simulink model "Modelo_Discreto_SS"  (R2019a)
settings: Solver=VariableStepAuto  StartTime=0.0  StopTime=500  RelTol=1e-3
model workspace (MAT data in the model file):
  P = [0.118997681558  0.340385726666  0.751267059306; 0.498364051982  0.58526775098  0.255095115459; 0.959743958516  0.223811939491  0.505957051665]
  xe = [0; 0; 0]
undefined symbols (not defined in the file or in its folder): sigbuilder_block
libraries: simulink x4
settings Model: OrderedModelArguments=off  Creator=Steven  LastModifiedBy=PC-88464
settings DataIOCC: ReturnWorkspaceOutputs=off
settings DebuggingCC: ArithmeticOperatorsInVariantConditions=warning
settings SFSimCC: SimUseLocalCustomCode=off
settings RTWCC: RTWUseLocalCustomCode=off
settings CodeAppCC: StateflowObjectComments=on

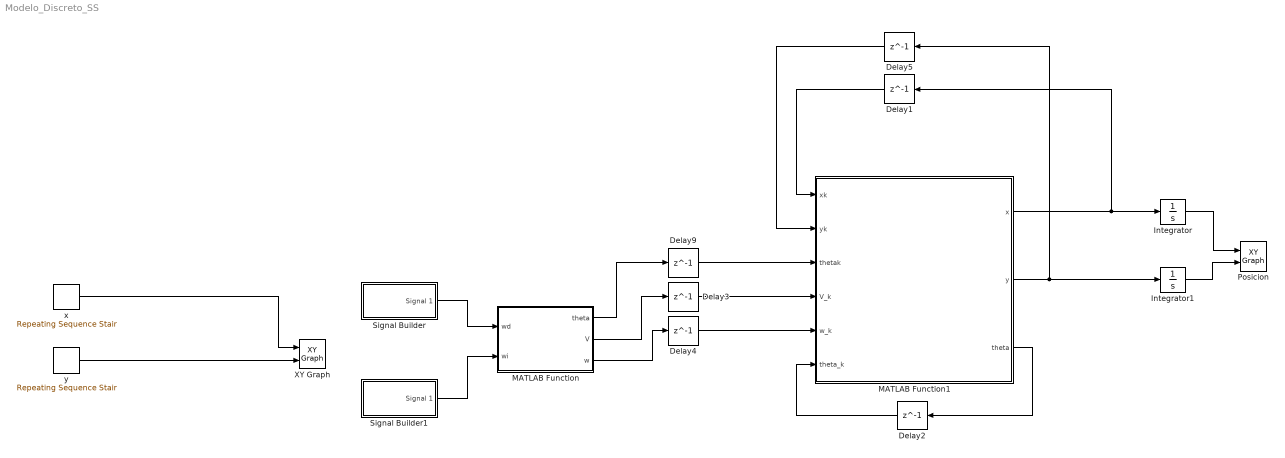
== system Modelo_Discreto_SS ==
  Delay{1..5,9} (6 alike) : Delay  DelayLength=1  InitialCondition=0  SampleTime=0.5
  Integrator : Integrator
  Integrator1 : Integrator
  MATLAB Function : MATLAB Function  TreatAsAtomicUnit=on
  MATLAB Function1 : MATLAB Function  TreatAsAtomicUnit=on  SystemSampleTime=0.5
  Posicion : simulink/Sinks/XY Graph  xmin=-2000  xmax=2000  ymin=-200  ymax=200  st=0.5
  Signal Builder : Subsystem  Tag=STV Subsys  LoadFcn=sigbuilder_block('load',[6 99 1012.5 413.25 ]);  StartFcn=sigbuilder_block('start');  StopFcn=sigbuilder_block('stop');  ClipboardFcn=sigbuilder_block('clipboard');  mask(Sigbuilder block){tuvar=[0:10]}
      mask help: Simulink:masks:SigbuilderBlock_MD
      mask init:
      | if ~strcmp(get_param(bdroot(gcbh),'SimulationStatus'),'stopped') tuvar = sigbuilder_block('maskInit'); end
      settings: CopyFcn=sigbuilder_block('copy');  DeleteFcn=sigbuilder_block('delete');  ModelCloseFcn=sigbuilder_block('modelClose');  PreSaveFcn=sigbuilder_block('preSave');  PauseFcn=sigbuilder_block('pause');  ContinueFcn=sigbuilder_block('continue');  NameChangeFcn=sigbuilder_block('namechange');  OpenFcn=sigbuilder_block('open',[51 123.75 1012.5 453.75 ]);  CloseFcn=sigbuilder_block('close');
      mask Display: plot(0, 0, 100, 100,[2, 2, 32, 32, 2], [68, 8, 8, 68, 68],[32, 2], [38, 38], [32, 19, 2],[53, 60, 44], [32, 17, 17, 2],[16, 16, 31, 31]);txt = getActiveGroup(gcbh);text(2, 100, txt,'verticalAlignment', 'top');
  Signal Builder1 : Subsystem  Tag=STV Subsys  LoadFcn=sigbuilder_block('load',[0.75 0.75 510.75 487.5 ]);  StartFcn=sigbuilder_block('start');  StopFcn=sigbuilder_block('stop');  ClipboardFcn=sigbuilder_block('clipboard');  mask(Sigbuilder block){tuvar=[0:10]}
      mask help: Simulink:masks:SigbuilderBlock_MD
      mask init:
      | if ~strcmp(get_param(bdroot(gcbh),'SimulationStatus'),'stopped') tuvar = sigbuilder_block('maskInit'); end
      settings: CopyFcn=sigbuilder_block('copy');  DeleteFcn=sigbuilder_block('delete');  ModelCloseFcn=sigbuilder_block('modelClose');  PreSaveFcn=sigbuilder_block('preSave');  PauseFcn=sigbuilder_block('pause');  ContinueFcn=sigbuilder_block('continue');  NameChangeFcn=sigbuilder_block('namechange');  OpenFcn=sigbuilder_block('open',[0.75 0.75 510.75 487.5 ]);  CloseFcn=sigbuilder_block('close');
      mask Display: plot(0, 0, 100, 100,[2, 2, 32, 32, 2], [68, 8, 8, 68, 68],[32, 2], [38, 38], [32, 19, 2],[53, 60, 44], [32, 17, 17, 2],[16, 16, 31, 31]);txt = getActiveGroup(gcbh);text(2, 100, txt,'verticalAlignment', 'top');
  XY Graph : simulink/Sinks/XY Graph  xmin=0  xmax=3000  ymin=0  ymax=200  st=-1
  x : simulink/Sources/Repeating Sequence Stair  OutValues="[0\t0\t0.122357536764706\t0.367004790785897\t0.733670540416495\t1.22188038737213\t1.83095716997706\t2.56002156384211\t3.40799286951678\t4.37358998651249\t5.45533257294931\t6.65154238993406\t7.96034482963452\t9.37967062587108\t10.9072577459058\t12.5074870935543\t14.1358531150623\t15.8024628907078\t17.5073781191743\t19.2506527356775\t21.0323328948846\t22.8524569547695\t24.6870589097060\t26.5315151793224\t28.3858216367550\t30.2499741436157\t32.1239685499954\t34.0078006944664\t35.9014664040855\t37.8049614943969\t39.7182817694354\t41.6414230217288\t43.5743810323012\t45.5171515706758\t47.4697303948779\t49.4321132514379\t51.4042958753942\t53.3862739902961\t55.3780433082071\t57.3795995297073\t59.3909383438971\t61.4055696132564\t63.4219031302490\t65.4399669647606\t67.4597607181438\t69.4812839897551\t71.5045363769553\t73.5295174751090\t75.5562268775849\t77.5846641757556\t79.6148289589977\t81.6467208146913\t83.6803393282207\t85.7156840829737\t87.7527546603420\t89.7915506397209\t91.8320715985093\t93.8743171121099\t95.9182867539287\t97.9639800953755\t100.011396705863\t102.060536152809\t104.111398001634\t106.163981815760\t108.218287156615\t110.274313583629\t112.332060654236\t114.391527923875\t116.452714945984\t118.515621272008\t120.580246451394\t122.646590031593\t124.714651558058\t126.784430574247\t128.855926621619\t130.929139239639\t133.004067965774\t135.080712335492\t137.158165631481\t139.236007260900\t141.314357332021\t143.393212510345\t145.472569461069\t147.552424849093\t149.632775339029\t151.713617595199\t153.794948281646\t155.876764062139\t157.959061600174\t160.041837558984\t162.125088601545\t164.208811390574\t166.293002588544\t168.377658857682\t170.464381318496\t172.559887389926\t174.665364252126\t176.780788702565\t178.906137065155\t181.041385190412\t183.186508455626\t185.341481765036\t187.506279550034\t189.680875769373\t191.865243909392\t194.059356984253\t196.263187536199\t198.476707635817\t200.699888882319\t202.932702403840\t205.175118857747\t207.427108430960\t209.688640840289\t211.959685332792\t214.240210686133\t216.530185208965\t218.829576741323\t221.138352655036\t223.456479854140\t225.783924775322\t228.120653388368\t230.466631196624\t232.821823237478\t235.186194082848\t237.559707839693\t239.942328150527\t242.334018193960\t244.734740685241\t247.144457876820\t249.563131558928\t251.990723060165\t254.427193248103\t256.872502529903\t259.326610852953\t261.789477705505\t264.261062117343\t266.741322660450\t269.230217449702\t271.727704143563\t274.232046667936\t276.742718200392\t279.259673024817\t281.782881593960\t284.312314136675\t286.847940658273\t289.389730940879\t291.937654543790\t294.491680803839\t297.051778835767\t299.617917532590\t302.190065565984\t304.768191386664\t307.352263224769\t309.942249090257\t312.538116773301\t315.139833844686\t317.747367656218\t320.360685341132\t322.979753814503\t325.602210367067\t328.226540419056\t330.852775638693\t333.480904426744\t336.110915157894\t338.742796180804\t341.376535818161\t344.012122366726\t346.649544097392\t349.288789255231\t351.929846059549\t354.572702703939\t357.217347356331\t359.863768159047\t362.511953228854\t365.161890657017\t367.813568509353\t370.466974826281\t373.122097622883\t375.778924888951\t378.437444589045\t381.097644662546\t383.759513023712\t386.423037561730\t389.088206140775\t391.755006600062\t394.423426753900\t397.093454391753\t399.765077278290\t402.438283153445\t405.113059732469\t407.789394705991\t410.467275740071\t413.146690476255\t415.827626531639\t418.510071498918\t421.194012946447\t423.879438418298\t426.566335434317\t429.254691490182\t431.944494057461\t434.635730583670\t437.328388492331\t440.019971324215\t442.711136014605\t445.401882563821\t448.092210972187\t450.782121240025\t453.471613367657\t456.160687355406\t458.849343203594\t461.537580912543\t464.225400482577\t466.912801914016\t469.599785207185\t472.286350362405\t474.972497379999\t477.658226260290\t480.343537003599\t483.028429610250\t485.712904080565\t488.396960414867\t491.080598613479\t493.763818676722\t496.446620604920\t499.129004398396\t501.810970057471\t504.492517582469\t507.173646973713\t509.854358231525\t512.534651356227\t515.214526348144\t517.893983207596\t520.573021934908\t523.251642530403\t525.929844994401\t528.607629327228\t531.284995529205\t533.961943600656\t536.638473541903\t539.314585353270\t541.990279035078\t544.665554587652\t547.340412011314\t550.014851306386\t552.688872473193\t555.362475512057\t558.035660423302\t560.708427207249\t563.380775864222\t566.052706394545\t568.724218798540\t571.395313076530\t574.065989228839\t576.736247255790\t579.406087157706\t582.075508934909\t584.744512587724\t587.413098116474\t590.081265521480\t592.749014803068\t595.416345961560\t598.083258997280\t600.749753910550\t603.415830701694\t606.081489371035\t608.746729918897\t611.411552345603\t614.075956651476\t616.739942836840\t619.403510902018\t622.066660847334\t624.729392673110\t627.391706379671\t630.053601967340\t632.715079436441\t635.371426414279\t638.023192098370\t640.670366275308\t643.312938777104\t645.950899481227\t648.584238310635\t651.212945233817\t653.837010264829\t656.456423463328\t659.071174934611\t661.681254829651\t664.286653345129\t666.887360723475\t669.483367252899\t672.074663267429\t674.661239146942\t677.243085317204\t679.820192249901\t682.392550462671\t684.960150519145\t687.522983028971\t690.081038647858\t692.634308077599\t695.182782066111\t697.726451407466\t700.265306941922\t702.799339555956\t705.328540182296\t707.852899799954\t710.372409434256\t712.887060156872\t715.396843085852\t717.901749385650\t720.401770267161\t722.896896987747\t725.387120851269\t727.872433208116\t730.352825455234\t732.828289036160\t735.298815441043\t737.764396206681\t740.225022916543\t742.680687200804\t745.131380736366\t747.577095246891\t750.017822502830\t752.453554321444\t754.884282566836\t757.309999149977\t759.730696028735\t762.146365207895\t764.556998739194\t766.962588721338\t769.363127300036\t771.758606668020\t774.149019065072\t776.534356778050\t778.914612140912\t781.289777534740\t783.659845387765\t786.024808175390\t788.384658420218\t790.739388692070\t793.088991608010\t795.433459832372\t797.772786076777\t800.106963100160\t802.435983708792\t804.759840756298\t807.078527143685\t809.392035819360\t811.700359779151\t814.003492066330\t816.301425771634\t818.594154033284\t820.881670037009\t823.163967016060\t825.441038251236\t827.712877070901\t829.979476851005\t832.240831015101\t834.496933034367\t836.747776427620\t838.993354761341\t841.233661649688\t843.468690754517\t845.698435785398\t847.922890499635\t850.142048702278\t852.355904246149\t854.564451031849\t856.767683007783\t858.965594170169\t861.158178563061\t863.345430278360\t865.527343455830\t867.703912283119\t869.875130995764\t872.040993877215\t874.201495258847\t876.356629519972\t878.506391087856\t880.650774437730\t882.789774092807\t884.923384624296\t887.051600651408\t889.174416841380\t891.291827909477\t893.403828619012\t895.510413781356\t897.611578255946\t899.707316950305\t901.797624820045\t903.882496868884\t905.961928148655\t908.035913759316\t910.104448848961\t912.167528613832\t914.225148298327\t916.277303195010\t918.323988644622\t920.365200036088\t922.400932806527\t924.431182441265\t926.455944473834\t928.475214485991\t930.488988107718\t932.497261017235\t934.500028941004\t936.497287653740\t938.489032978414\t940.475260786263\t942.455966996795\t944.431147577798\t946.400798545341\t948.364915963785\t950.323495945786\t952.276534652301\t954.224028292595\t956.170911904799\t958.117630417913\t960.064183812303\t962.010572068341\t963.956795166400\t965.902853086859\t967.848745810101\t969.794473316515\t971.740035586491\t973.685432600425\t975.630664338719\t977.575730781776\t979.520631910005\t981.465367703820\t983.409938143637\t985.354343209879\t987.298582882972\t989.242657143345\t991.186565971434\t993.130309347677\t995.073887252517\t997.017299666402\t998.960546569784\t1000.90362794312\t1002.84654376686\t1004.78929402149\t1006.73187868746\t1008.67429774524\t1010.61655117533\t1012.55863895819\t1014.50056107432\t1016.44231750420\t1018.38390822833\t1020.32533322721\t1022.26659248134\t1024.20768597123\t1026.14861367738\t1028.08937558033\t1030.02997166058\t1031.97040189866\t1033.91066627510\t1035.85076477043\t1037.79069736519\t1039.73046403992\t1041.67006477518\t1043.60949955150\t1045.54876834944\t1047.48787114956\t1049.42680793243\t1051.36557867861\t1053.30418336868\t1055.24262198320\t1057.18089450276\t1059.11900090795\t1061.05694117935\t1062.99471529756\t1064.93232324318\t1066.86976499680\t1068.80704053903\t1070.74414985048\t1072.68109291177\t1074.61786970352\t1076.55448020634\t1078.49092440087\t1080.42720226774\t1082.36331378759\t1084.29925894105\t1086.23503770877\t1088.17065007139\t1090.10609600958\t1092.04137550399\t1093.97648853528\t1095.91143508412\t1097.84621513117\t1099.78082865712\t1101.71527564264\t1103.64955606841\t1105.58366991512\t1107.51761716347\t1109.45139779415\t1111.38501178786\t1113.31845912531\t1115.25173978720\t1117.18485375425\t1119.11780100718\t1121.05058152670\t1122.98319529355\t1124.91564228845\t1126.84792249215\t1128.78003588537\t1130.71198244886\t1132.64376216337\t1134.57537500966\t1136.50682096847\t1138.43810002057\t1140.36921214673\t1142.30015732771\t1144.23093554428\t1146.16154677723\t1148.09199100734\t1150.02226821539\t1151.95237838218\t1153.88232148849\t1155.81209751513\t1157.74170644290\t1159.67114825262\t1161.60042292508\t1163.52953044112\t1165.45847078154\t1167.38724392718\t1169.31584985886\t1171.24428855742\t1173.17256000369\t1175.10066417853\t1177.02860106276\t1178.95637063726\t1180.88397288286\t1182.81140778044\t1184.73867531085\t1186.66577545496\t1188.59270819364\t1190.51947350778\t1192.44607137825\t1194.37250178594\t1196.29876471174\t1198.22486013654\t1200.15078804123\t1202.07654840673\t1204.00214121394\t1205.92756644378\t1207.85282407714\t1209.77791409496\t1211.70283647817\t1213.62759120768\t1215.55217826443\t1217.47659762936\t1219.40084928341\t1221.32493320752\t1223.24884938265\t1225.17259778975\t1227.09617840978\t1229.01959122369\t1230.94283621247\t1232.86591335707\t1234.78882263848\t1236.71156403767\t1238.63413753563\t1240.55654311335\t1242.47878075183\t1244.40085043205\t1246.32275213502\t1248.24448584174\t1250.16605153323\t1252.08744919051\t1254.00867879458\t1255.92974032647\t1257.85063376722\t1259.77135909785\t1261.69191629939\t1263.61230535289\t1265.53252623940\t1267.45257893996\t1269.37246343562\t1271.29217970745\t1273.21172773650\t1275.13110750384\t1277.05031899054\t1278.96936217768\t1280.88823704634\t1282.80694357760\t1284.72548175254\t1286.64385155226\t1288.56205295786\t1290.48008595043\t1292.39795051109\t1294.31564662093\t1296.23317426108\t1298.15053341266\t1300.06772405677\t1301.98474617456\t1303.90159974716\t1305.81828475568\t1307.73480118129\t1309.65114900512\t1311.56732820831\t1313.48333877203\t1315.39918067743\t1317.31485390566\t1319.23035843790\t1321.14569425532\t1323.06086133908\t1324.97585967038\t1326.89068923038\t1328.80535000028\t1330.71984196126\t1332.63416509453\t1334.54831938129\t1336.46230480273\t1338.37612134007\t1340.28976897452\t1342.20324768730\t1344.11655745962\t1346.02969827272\t1347.94267010783\t1349.85547294617\t1351.76810676899\t1353.68057155754\t1355.59286729305\t1357.50499395678\t1359.41695152998\t1361.32873999393\t1363.24035932987\t1365.15180951909\t1367.06309054285\t1368.97420238243\t1370.88514501912\t1372.79591843419\t1374.70652260895\t1376.61695752468\t1378.52722316269\t1380.43731950427\t1382.34724653074\t1384.25700422341\t1386.16659256360\t1388.07601153262\t1389.98526111180\t1391.89434128247\t1393.80325202597\t1395.71199332363\t1397.62056515680\t1399.52896750682\t1401.43720035504\t1403.34526368282\t1405.25315747152\t1407.16088170250\t1409.06843635713\t1410.97582141679\t1412.88303686285\t1414.79008267669\t1416.69695883970\t1418.60366533326\t1420.51020213878\t1422.41656923765\t1424.32276661128\t1426.22879424106\t1428.13465210842\t1430.04034019477\t1431.94585848153\t1433.85120695012\t1435.75638558198\t1437.66139435853\t1439.56623326122\t1441.47090227148\t1443.37540137077\t1445.27973054052\t1447.18388976221\t1449.08787901728\t1450.99169828721\t1452.89534755345\t1454.79882679749\t1456.70213600079\t1458.60527514484\t1460.50824421112\t1462.41104318113\t1464.31367203635\t1466.21613075829\t1468.11841932845\t1470.02053772833\t1471.92248593945\t1473.82426394332\t1475.72587172146\t1477.62730925540\t1479.52857652666\t1481.42967351677\t1483.33060020728\t1485.23135657973\t1487.13194261566\t1489.03235829662\t1490.93260360416\t1492.83267851985\t1494.73258302525\t1496.63231710192\t1498.53188073144\t1500.43127389539\t1502.33049657533\t1504.22954875287\t1506.12843040958\t1508.02714152707\t1509.92568208692\t1511.82405207075\t1513.72225146015\t1515.62028023675\t1517.51813838214\t1519.41582587796\t1521.31334270583\t1523.21068884737\t1525.10786428421\t1527.00486899801\t1528.90170297039\t1530.79836618299\t1532.69485861749\t1534.59118025551\t1536.48733107873\t1538.38331106880\t1540.27912020740\t1542.17475847619\t1544.07022585686\t1545.96552233107\t1547.86064788052\t1549.75560248689\t1551.65038613188\t1553.54499879719\t1555.43944046451\t1557.33371111556\t1559.22781073203\t1561.12173929566\t1563.01549678815\t1564.90908319124\t1566.80249848664\t1568.69574265610\t1570.58881568134\t1572.48171754411\t1574.37444822615\t1576.26700770922\t1578.15939597506\t1580.05161300544\t1581.94365878211\t1583.83553328685\t1585.72723650143\t1587.61876840762\t1589.51012898720\t1591.40131822195\t1593.29233609367\t1595.18318258414\t1597.07385767517\t1598.96436134856\t1600.85469358611\t1602.74485436963\t1604.63484368094\t1606.52466150185\t1608.41430781419\t1610.30378259979\t1612.19308584048\t1614.08221751809\t1615.97117761447\t1617.85996611146\t1619.74858299091\t1621.63702823468\t1623.52530182462\t1625.41340374259\t1627.30133397046\t1629.18909249010\t1631.07667928340\t1632.96409433222\t1634.85133761845\t1636.73840912398\t1638.62530883070\t1640.51203672052\t1642.39859277533\t1644.28497697703\t1646.17118930754\t1648.05722974877\t1649.94309828265\t1651.82879489109\t1653.71431955602\t1655.59967225937\t1657.48485298308\t1659.36986170910\t1661.25469841936\t1663.13936309581\t1665.02385572042\t1666.90817627512\t1668.79232474190\t1670.67630110272\t1672.56010533953\t1674.44373743434\t1676.32719736910\t1678.21048512581\t1680.09360068645\t1681.97654403302\t1683.85931514751\t1685.74191401193\t1687.62434060828\t1689.50659491857\t1691.38867692481\t1693.27058660903\t1695.15232395325\t1697.03388893949\t1698.91528154979\t1700.79650176619\t1702.67754957072\t1704.55842494542\t1706.43912787236\t1708.31965833358\t1710.20001631113\t1712.08020178709\t1713.96021474352\t1715.84005516249\t1717.71972302607\t1719.59921831635\t1721.47854101541\t1723.35769110534\t1725.23666856822\t1727.11547338617\t1728.99410554127\t1730.87256501564\t1732.75085179138\t1734.62896585062\t1736.50690717546\t1738.38467574803\t1740.26227155047\t1742.13969456489\t1744.01694477345\t1745.89402215827\t1747.77092670150\t1749.64765838530\t1751.52421719182\t1753.40060310321\t1755.27681610163\t1757.15285616927\t1759.02872328827\t1760.90441744083\t1762.77993860912\t1764.65528677532\t1766.53046192163\t1768.40546403023\t1770.28029308333\t1772.15494906312\t1774.02943195182\t1775.90374173162\t1777.77787838475\t1779.65184189343\t1781.52563223988\t1783.39924940632\t1785.27269337499\t1787.14596412813\t1789.01906164797\t1790.89198591677\t1792.76473691676\t1794.63731463021\t1796.50971903938\t1798.38195012652\t1800.25400787390\t1802.12589226380\t1803.99760327848\t1805.86914090024\t1807.74050511135\t1809.61169589411\t1811.48271323080\t1813.35355710372\t1815.22422749518\t1817.09472438748\t1818.96504776294\t1820.83519760386\t1822.70517389257\t1824.57497661139\t1826.44460574265\t1828.31406126868\t1830.18334317182\t1832.05245143441\t1833.92138603879\t1835.79014696731\t1837.65873420233\t1839.52714772621\t1841.39538752131\t1843.26345357000\t1845.13134585465\t1846.99906435763\t1848.86660906132\t1850.73397994812\t1852.60117700040\t1854.46820020057\t1856.33504953102\t1858.20172497415\t1860.06822651237\t1861.93455412809\t1863.80070780372\t1865.66668752169\t1867.53249326442\t1869.39812501433\t1871.26358275387\t1873.12886646546\t1874.99397613155\t1876.85891173458\t1878.72367325701\t1880.58826068129\t1882.45267398988\t1884.31691316524\t1886.18097818983\t1888.04486904614\t1889.90858571664\t1891.77212818380\t1893.63549643012\t1895.49869043807\t1897.36171019017\t1899.22455566890\t1901.08722685677\t1902.94972373628\t1904.81204628995\t1906.67419450029\t1908.53616834982\t1910.39796782106\t1912.25959289656\t1914.12104355882\t1915.98231979041\t1917.84342157385\t1919.70434889169\t1921.56510172649\t1923.42568006080\t1925.28608387717\t1927.14631315818\t1929.00636788639\t1930.86624804437\t1932.72595361470\t1934.58548457997\t1936.44484092274\t1938.30402262563\t1940.16302967121\t1942.02186204210\t1943.88051972088\t1945.73900269018\t1947.59731093260\t1949.45544443076\t1951.31340316727\t1953.17118712477\t1955.02879628588\t1956.88623063324\t1958.74349014948\t1960.60057481725\t1962.45748461919\t1964.31421953795\t1966.17077955620\t1968.02716465659\t1969.88337482178\t1971.73941003444\t1973.59527027725\t1975.45095553289\t1977.30646578403\t1979.16180101336\t1981.01696120357\t1982.87194633736\t1984.72675639742\t1986.58139136647\t1988.43585122720\t1990.29013596233\t1992.14424555458\t1993.99817998667\t1995.85193924132\t1997.70552330126\t1999.55893214924\t2001.41216576797\t2003.26522414022\t2005.11810724873\t2006.97081507624\t2008.82334760551\t2010.67570481932\t2012.52788670041\t2014.37989323156\t2016.23172439554\t2018.08338017514\t2019.93486055313\t2021.78616551229\t2023.63729503543\t2025.48824910534\t2027.33902770481\t2029.18963081665\t2031.04005842368\t2032.89031050869\t2034.74038705452\t2036.59028804398\t2038.44001345989\t2040.28956328510\t2042.13893750242\t2043.98813609472\t2045.83715904481\t2047.68600633556\t2049.53467794982\t2051.38317387045\t2053.23149408029\t2055.07963856223\t2056.92760729913\t2058.77540027387\t2060.62301746931\t2062.47045886836\t2064.31772445389\t2066.16481420879\t2068.01172811597].'"  tsamp=-1  OutMin=[]  OutMax=[]  OutDataTypeStr=double  OutputDataTypeScalingMode=double  OutDataType=fixdt(0,8)  ConRadixGroup=Best Precision: Vector-wise  OutScaling=2^-12
  y : simulink/Sources/Repeating Sequence Stair  OutValues="[0\t0\t0\t0.00576092982047422\t0.0230389295880498\t0.0575789670167764\t0.115108463536273\t0.201330934567526\t0.321919649236809\t0.482511314804011\t0.688699791063534\t0.946029839953929\t1.25999091558661\t1.63601099987418\t2.07945048890546\t2.58511571301662\t3.11890223099872\t3.64946310464757\t4.17618168427347\t4.69844004811736\t5.21561909015051\t5.72709860807187\t6.22573523578382\t6.72827450597351\t7.23472878793874\t7.74511044736462\t8.25943184631406\t8.77770534321823\t9.29994329286710\t9.82615804639984\t10.3563619512954\t10.8905673513630\t11.4287865867324\t11.9710319938448\t12.5173159054431\t13.0676506505622\t13.6220485545200\t14.1805219389074\t14.7430831215792\t15.3097444166444\t15.8805181344567\t16.4535717181467\t17.0257539278886\t17.5969626292051\t18.1671957554319\t18.7364512400015\t19.3047270164448\t19.8720210183929\t20.4383311795788\t21.0036554338393\t21.5679917151165\t22.1313379574598\t22.6936920950276\t23.2550520620887\t23.8154157930247\t24.3747812223311\t24.9331462846195\t25.4905089146193\t26.0468670471790\t26.6022186172686\t27.1565615599809\t27.7098938105334\t28.2622133042701\t28.8135179766632\t29.3638057633147\t29.9130745999585\t30.4613224224617\t31.0085471668270\t31.5547467691935\t32.0999191658395\t32.6440622931834\t33.1871740877860\t33.7292524863520\t34.2702954257317\t34.8103008429232\t35.3492666750733\t35.8871908594802\t36.4240713335945\t36.9596723889130\t37.4931198405867\t38.0239346738456\t38.5521164504276\t39.0776647362932\t39.6005791016250\t40.1208591208280\t40.6385043725300\t41.1535144395807\t41.6658889090530\t42.1756273722420\t42.6827294246654\t43.1871946660637\t43.6890227004001\t44.1882131358604\t44.6847655848530\t45.1790597214688\t45.6713277120772\t46.1564127518179\t46.6342382907423\t47.1047278463799\t47.5678050063942\t48.0233934312373\t48.4714168568052\t48.9117990970928\t49.3444640468484\t49.7693356842277\t50.1863380734473\t50.5953953674385\t50.9964318104993\t51.3893717409465\t51.7741395937669\t52.1506599032674\t52.5188573057247\t52.8786565420340\t53.2299824603557\t53.5727600187627\t53.9069142878849\t54.2323704535534\t54.5490538194432\t54.8568898097141\t55.1558039716512\t55.4457219783020\t55.7265696311143\t55.9982728625702\t56.2607577388195\t56.5139504623116\t56.7577773744244\t56.9921649580919\t57.2170398404302\t57.4323287953600\t57.6379587462287\t57.8338567684287\t58.0199500920143\t58.1961661043159\t58.3624323525518\t58.5186765464372\t58.6648265607909\t58.8008104381396\t58.9265563913184\t59.0419928060697\t59.1469772598390\t59.2430081924803\t59.3304343609552\t59.4092128428218\t59.4793008173064\t59.5406555663462\t59.5932344756315\t59.6369950356453\t59.6718948427032\t59.6978915999911\t59.7149431186016\t59.7230073185695\t59.7220422299060\t59.7120059936309\t59.6928568628041\t59.6645532035559\t59.6270534961145\t59.5803163358342\t59.5243004342202\t59.4589646199533\t59.3843341307166\t59.3026920653126\t59.2155344328683\t59.1228529737864\t59.0246394528773\t58.9208856594316\t58.8115834072928\t58.6967245349296\t58.5763009055083\t58.4503044069650\t58.3187269520777\t58.1815604785384\t58.0387969490251\t57.8904283512731\t57.7364466981474\t57.5768440277137\t57.4116124033099\t57.2407439136178\t57.0642306727340\t56.8820648202411\t56.6942385212787\t56.5007439666142\t56.3015733727137\t56.0967189818126\t55.8861730619861\t55.6699279072196\t55.4479758374790\t55.2203091987810\t54.9869203632628\t54.7478017292526\t54.5029457213390\t54.2523447904406\t53.9959914138762\t53.7338780954335\t53.4659973654389\t53.1923417808266\t52.9129039252079\t52.6276764089395\t52.3366518691933\t52.0398229700243\t51.7371824024398\t51.4287228844674\t51.1144371612236\t50.7946131464463\t50.4748289760865\t50.1550846531553\t49.8353801806641\t49.5157155616243\t49.1960907990470\t48.8765058959435\t48.5569608553251\t48.2374556802031\t47.9179903735888\t47.5985649384934\t47.2791793779283\t46.9598336949045\t46.6405278924335\t46.3212619735265\t46.0020359411948\t45.6828497984496\t45.3637035483021\t45.0445971937637\t44.7255307378455\t44.4065041835589\t44.0875175339151\t43.7685707919253\t43.4496639606007\t43.1307970429527\t42.8119700419925\t42.4931829607312\t42.1744358021803\t41.8557285693507\t41.5370612652540\t41.2184338929011\t40.8998464553035\t40.5812989554722\t40.2627913964187\t39.9443237811539\t39.6258961126893\t39.3075083940360\t38.9891606282053\t38.6708528182083\t38.3525849670563\t38.0343570777604\t37.7161691533320\t37.3980211967822\t37.0799132111223\t36.7618451993633\t36.4438171645167\t36.1258291095934\t35.8078810376049\t35.4899729515621\t35.1721048544765\t34.8542767493591\t34.5364886392211\t34.2187405270738\t33.9010324159283\t33.5833643087959\t33.2657362086877\t32.9481481186148\t32.6306000415886\t32.3130919806201\t31.9956239387206\t31.6781959189012\t31.3608079241731\t31.0434599575475\t30.7261520220356\t30.4088841206485\t30.0916562563974\t29.7744684322935\t29.4573206513479\t29.1402129165718\t28.8231452309764\t28.5061175975729\t28.1891300193723\t27.8721824993858\t27.5558362404931\t27.2447373513668\t26.9388688407777\t26.6382136978499\t26.3427548921681\t26.0524753738840\t25.7673580738237\t25.4873859035946\t25.2125417556928\t24.9428085036100\t24.6781690019411\t24.4186060864916\t24.1641025743847\t23.9146412641691\t23.6702049359267\t23.4307763513797\t23.1963382539988\t22.9668733691110\t22.7423644040071\t22.5227940480495\t22.3081449727810\t22.0983998320316\t21.8935412620278\t21.6935518814998\t21.4984142917901\t21.3081110769621\t21.1226248039077\t20.9419380224563\t20.7660332654829\t20.5948930490169\t20.4284998723504\t20.2668362181470\t20.1098845525504\t19.9576273252931\t19.8100469698053\t19.6671259033237\t19.5288465270005\t19.3951912260122\t19.2661423696686\t19.1416823115222\t19.0217933894769\t18.9064579258974\t18.7956582277184\t18.6893765865539\t18.5875952788064\t18.4902965657766\t18.3974626937724\t18.3090758942188\t18.2251183837670\t18.1455723644044\t18.0704200235640\t17.9996435342340\t17.9332250550678\t17.8711467304935\t17.8133906908240\t17.7599390523665\t17.7107739175327\t17.6658773749486\t17.6252314995646\t17.5888183527654\t17.5566199824803\t17.5286184232931\t17.5047956965524\t17.4851338104819\t17.4696147602903\t17.4582205282819\t17.4509330839670\t17.4477343841719\t17.4486063731498\t17.4535309826907\t17.4624901322323\t17.4754657289705\t17.4924396679698\t17.5133938322738\t17.5383100930163\t17.5671703095314\t17.5999563294646\t17.6366499888834\t17.6772331123881\t17.7216875132226\t17.7699949933852\t17.8221373437396\t17.8780963441256\t17.9378537634702\t18.0013913598987\t18.0686908808453\t18.1397340631645\t18.2145026332418\t18.2929783071053\t18.3751427905364\t18.4609777791810\t18.5504649586608\t18.6435860046845\t18.7403225831588\t18.8406563502999\t18.9445689527447\t19.0520420276621\t19.1630572028643\t19.2775960969183\t19.3956403192568\t19.5171714702904\t19.6421711415181\t19.7706209156395\t19.9025023666659\t20.0377970600318\t20.1764865527065\t20.3185523933055\t20.4639761222022\t20.6127392716393\t20.7648233658405\t20.9202099211221\t21.0788804460044\t21.2408164413237\t21.4059994003436\t21.5744108088669\t21.7460321453471\t21.9208448810004\t22.0988304799169\t22.2799703991728\t22.4642460889419\t22.6516389926075\t22.8421305468738\t23.0357021818782\t23.2323353213027\t23.4320113824858\t23.6347117765343\t23.8404179084351\t24.0491111771672\t24.2607729758132\t24.4753846916714\t24.6929277063676\t24.9133833959668\t25.1367331310853\t25.3629582770023\t25.5920401937721\t25.8239602363357\t26.0586997546327\t26.2962400937134\t26.5365625938504\t26.7802668102704\t27.0237741154373\t27.2670845407212\t27.5101981174940\t27.7531148771295\t27.9958348510035\t28.2383580704937\t28.4806845669797\t28.7228143718431\t28.9647475164674\t29.2064840322381\t29.4480239505424\t29.6893673027698\t29.9305141203113\t30.1714644345603\t30.4122182769117\t30.6527756787627\t30.8931366715120\t31.1333012865607\t31.3732695553114\t31.6130415091690\t31.8526171795401\t32.0919965978332\t32.3311797954589\t32.5701668038296\t32.8089576543596\t33.0475523784653\t33.2859510075648\t33.5241535730782\t33.7621601064276\t33.9999706390369\t34.2375852023321\t34.4750038277410\t34.7122265466932\t34.9492533906205\t35.1860843909563\t35.4227195791362\t35.6591589865976\t35.8954026447799\t36.1314505851241\t36.3673028390735\t36.6029594380732\t36.8384204135702\t37.0736857970133\t37.3087556198534\t37.5436299135432\t37.7783087095373\t38.0127920392923\t38.2470799342667\t38.4811724259208\t38.7150695457169\t38.9487713251193\t39.1822777955941\t39.4155889886092\t39.6487049356347\t39.8816256681423\t40.1143512176057\t40.3468816155008\t40.5792168933049\t40.8113570824977\t41.0433022145604\t41.2750523209763\t41.5066074332307\t41.7379675828107\t41.9691328012051\t42.2001031199050\t42.4308785704031\t42.6614591841942\t42.8918449927748\t43.1220360276435\t43.3520323203006\t43.5818339022485\t43.8114408049914\t44.0408530600354\t44.2700706988886\t44.4990937530607\t44.7279222540637\t44.9565562334112\t45.1849957226189\t45.4132407532042\t45.6412913566865\t45.8691475645871\t46.0968094084293\t46.3242769197380\t46.5515501300402\t46.7786290708649\t47.0055137737428\t47.2322042702065\t47.4587005917906\t47.6850027700314\t47.9111108364674\t48.1370248226388\t48.3627447600876\t48.5882706803578\t48.8136026149954\t49.0387405955481\t49.2636846535655\t49.4884348205992\t49.7129911282027\t49.9373536079312\t50.1615222913420\t50.3854972099941\t50.6092783954486\t50.8328658792682\t51.0562596930177\t51.2794598682638\t51.5024664365750\t51.7252794295216\t51.9478988786759\t52.1703248156120\t52.3925572719061\t52.6145962791360\t52.8364418688815\t53.0580940727242\t53.2795529222478\t53.5008184490376\t53.7218906846810\t53.9427696607671\t54.1634554088870\t54.3839479606336\t54.6042473476018\t54.8243536013882\t55.0442667535913\t55.2639868358117\t55.4835138796515\t55.7028479167151\t55.9219889786083\t56.1409370969393\t56.3596923033177\t56.5782546293552\t56.7966241066653\t57.0148007668635\t57.2327846415671\t57.4505757623951\t57.6681741609685\t57.8855798689103\t58.1027929178452\t58.3198133393998\t58.5366411652026\t58.7532764268839\t58.9697191560759\t59.1859693844127\t59.4020271435303\t59.6178924650663\t59.8335653806606\t60.0490459219546\t60.2643341205916\t60.4794300082171\t60.6943336164779\t60.9090449770232\t61.1235641215038\t61.3378910815722\t61.5520258888832\t61.7659685750930\t61.9797191718600\t62.1932777108443\t62.4066442237078\t62.6198187421144\t62.8328012977297\t63.0455919222214\t63.2581906472588\t63.4705975045131\t63.6828125256575\t63.8948357423668\t64.1066671863181\t64.3183068891898\t64.5297548826625\t64.7410111984186\t64.9520758681423\t65.1629489235197\t65.3736303962386\t65.5841203179889\t65.7944187204621\t66.0045256353518\t66.2144410943531\t66.4241651291633\t66.6336977714815\t66.8430390530083\t67.0521890054466\t67.2611476605008\t67.4699150498773\t67.6784912052845\t67.8868761584322\t68.0950699410325\t68.3030725847991\t68.5108841214477\t68.7185045826955\t68.9259340002620\t69.1331724058681\t69.3402198312370\t69.5470763080934\t69.7537418681639\t69.9602165431770\t70.1665003648630\t70.3725933649540\t70.5784955751841\t70.7842070272891\t70.9897277530066\t71.1950577840760\t71.4001971522389\t71.6051458892382\t71.8099040268190\t72.0144715967281\t72.2188486307142\t72.4230351605278\t72.6270312179211\t72.8308368346484\t73.0344520424657\t73.2378768731306\t73.4411113584030\t73.6441555300442\t73.8470094198175\t74.0496730594881\t74.2521464808230\t74.4544297155909\t74.6565227955624\t74.8584257525099\t75.0601386182078\t75.2616614244321\t75.4629942029607\t75.6641369855733\t75.8650898040515\t76.0658526901786\t76.2664256757400\t76.4668087925225\t76.6670020723150\t76.8670055469083\t77.0668192480947\t77.2664432076686\t77.4658774574261\t77.6651220291651\t77.8641769546854\t78.0630422657885\t78.2617179942779\t78.4602041719588\t78.6585008306381\t78.8566080021248\t79.0545257182294\t79.2522540107645\t79.4497929115443\t79.6471424523850\t79.8443026651043\t80.0412735815221\t80.2380552334599\t80.4346476527410\t80.6310508711905\t80.8272649206355\t81.0232898329047\t81.2191256398288\t81.4147723732399\t81.6102300649725\t81.8054987468624\t82.0005784507476\t82.1954692084676\t82.3901710518638\t82.5846840127795\t82.7790081230597\t82.9731434145513\t83.1670899191028\t83.3608476685648\t83.5544166947895\t83.7477970296310\t83.9409887049451\t84.1339917525894\t84.3268062044235\t84.5194320923085\t84.7118694481076\t84.9041183036855\t85.0961786909091\t85.2880506416466\t85.4797341877684\t85.6712293611464\t85.8625361936547\t86.0536547171687\t86.2445849635660\t86.4353269647257\t86.6258807525289\t86.8162463588584\t87.0064238155989\t87.1964131546366\t87.3862144078599\t87.5758276071588\t87.7652527844249\t87.9544899715519\t88.1435392004352\t88.3324005029719\t88.5210739110609\t88.7095594566030\t88.8978571715008\t89.0859670876584\t89.2738892369820\t89.4616236513796\t89.6491703627607\t89.8365294030368\t90.0237008041212\t90.2106845979288\t90.3974808163766\t90.5840894913831\t90.7705106548686\t90.9567443387553\t91.1427905749673\t91.3286493954301\t91.5143208320713\t91.6998049168202\t91.8851016816079\t92.0702111583672\t92.2551333790326\t92.4398683755407\t92.6244161798296\t92.8087768238393\t92.9929503395114\t93.1769367587896\t93.3607361136190\t93.5443484359468\t93.7277737577219\t93.9110121108947\t94.0940635274177\t94.2769280392450\t94.4596056783326\t94.6420964766383\t94.8244004661213\t95.0065176787431\t95.1884481464666\t95.3701919012567\t95.5517489750798\t95.7331193999043\t95.9143032077003\t96.0953004304397\t96.2761111000960\t96.4567352486448\t96.6371729080631\t96.8174241103298\t96.9974888874258\t97.1773672713334\t97.3570592940369\t97.5365649875222\t97.7158843837772\t97.8950175147913\t98.0739644125558\t98.2527251090637\t98.4312996363099\t98.6096880262909\t98.7878903110051\t98.9659065224525\t99.1437366926349\t99.3213808535561\t99.4988390372212\t99.6761112756375\t99.8531976008138\t100.030098044761\t100.206812639491\t100.383341417018\t100.559684409358\t100.735841648529\t100.911813166550\t101.087598995443\t101.263199167229\t101.438613713935\t101.613842667586\t101.788886060210\t101.963743923837\t102.138416290500\t102.312903192231\t102.487204661066\t102.661320729042\t102.835251428196\t103.008996790570\t103.182556848207\t103.355931633148\t103.529121177442\t103.702125513134\t103.874944672273\t104.047578686912\t104.220027589102\t104.392291410898\t104.564370184356\t104.736263941534\t104.907972714491\t105.079496535289\t105.250835435991\t105.421989448662\t105.592958605368\t105.763742938177\t105.934342479160\t106.104757260389\t106.274987313936\t106.445032671878\t106.614893366291\t106.784569429254\t106.954060892847\t107.123367789153\t107.292490150255\t107.461428008240\t107.630181395194\t107.798750343207\t107.967134884370\t108.135335050775\t108.303350874517\t108.471182387691\t108.638829622396\t108.806292610731\t108.973571384798\t109.140665976698\t109.307576418538\t109.474302742423\t109.640844980462\t109.807203164764\t109.973377327441\t110.139367500607\t110.305173716377\t110.470796006867\t110.636234404196\t110.801488940484\t110.966559647853\t111.131446558428\t111.296149704332\t111.460669117694\t111.625004830642\t111.789156875307\t111.953125283822\t112.116910088319\t112.280511320936\t112.443929013809\t112.607163199078\t112.770213908883\t112.933081175367\t113.095765030675\t113.258265506952\t113.420582636347\t113.582716451008\t113.744666983088\t113.906434264738\t114.068018328114\t114.229419205372\t114.390636928669\t114.551671530166\t114.712523042025\t114.873191496407\t115.033676925479\t115.193979361407\t115.354098836359\t115.514035382505\t115.673789032016\t115.833359817068\t115.992747769833\t116.151952922490\t116.310975307217\t116.469814956194\t116.628471901603\t116.786946175627\t116.945237810453\t117.103346838267\t117.261273291258\t117.419017201617\t117.576578601535\t117.733957523207\t117.891153998828\t118.048168060596\t118.204999740709\t118.361649071368\t118.518116084775\t118.674400813135\t118.830503288654\t118.986423543538\t119.142161609998\t119.297717520244\t119.453091306488\t119.608283000944\t119.763292635830\t119.918120243362\t120.072765855759\t120.227229505244\t120.381511224038\t120.535611044366\t120.689528998454\t120.843265118530\t120.996819436823\t121.150191985565\t121.303382796988\t121.456391903328\t121.609219336819\t121.761865129701\t121.914329314213\t122.066611922596\t122.218712987093\t122.370632539949\t122.522370613410\t122.673927239725\t122.825302451142\t122.976496279914\t123.127508758294\t123.278339918536\t123.428989792897\t123.579458413636\t123.729745813011\t123.879852023284\t124.029777076719\t124.179521005580\t124.329083842135\t124.478465618651\t124.627666367398\t124.776686120648\t124.925524910674\t125.074182769751\t125.222659730155\t125.370955824166\t125.519071084063\t125.667005542127\t125.814759230642\t125.962332181893\t126.109724428166\t126.256936001750\t126.403966934936\t126.550817260014\t126.697487009278\t126.843976215022\t126.990284909545\t127.136413125143\t127.282360894118\t127.428128248771\t127.573715221404\t127.719121844324\t127.864348149836\t128.009394170250\t128.154259937875\t128.298945485024\t128.443450844008\t128.587776047144\t128.731921126748\t128.875886115138\t129.019671044635\t129.163275947560\t129.306700856236\t129.449945802989\t129.593010820145\t129.735895940032\t129.878601194980\t130.021126617322\t130.163472239390\t130.305638093519\t130.447624212047\t130.589430627310\t130.731057371649\t130.872504477406\t131.013771976924\t131.154859902548\t131.295768286624\t131.436497161501\t131.577046559528\t131.717416513056\t131.857607054440\t131.997618216034\t132.137450030194\t132.277102529278\t132.416575745647\t132.555869711661\t132.694984459683\t132.833920022079\t132.972676431214\t133.111253719458\t133.249651919178\t133.387871062747\t133.525911182537\t133.663772310924\t133.801454480283\t133.938957722992\t134.076282071430\t134.213427557980\t134.350394215023\t134.487182074944\t134.623791170130\t134.760221532967\t134.896473195846\t135.032546191156\t135.168440551292\t135.304156308647\t135.439693495616\t135.575052144599\t135.710232287993\t135.845233958200\t135.980057187622\t136.114702008663\t136.249168453730\t136.383456555228\t136.517566345568\t136.651497857160\t136.785251122416].'"  tsamp=-1  OutMin=[]  OutMax=[]  OutDataTypeStr=double  OutputDataTypeScalingMode=double  OutDataType=fixdt(0,8)  ConRadixGroup=Best Precision: Vector-wise  OutScaling=2^-12
  wires:
  MATLAB Function/2(V) -> Delay3/1
  MATLAB Function/3(w) -> Delay4/1
  Delay4/1 -> MATLAB Function1/5(w_k)
  Delay3/1 -> MATLAB Function1/4(V_k)
  MATLAB Function1/3(theta) -> Delay2/1
  Delay2/1 -> MATLAB Function1/6(theta_k)
  Delay1/1 -> MATLAB Function1/1(xk)
  Delay5/1 -> MATLAB Function1/2(yk)
  MATLAB Function1/1(x) -> Integrator/1, Delay1/1
  MATLAB Function1/2(y) -> Integrator1/1, Delay5/1
  MATLAB Function/1(theta) -> Delay9/1
  Delay9/1 -> MATLAB Function1/3(thetak)
  y/1 -> XY Graph/2
  x/1 -> XY Graph/1
  Integrator/1 -> Posicion/1
  Integrator1/1 -> Posicion/2
  Signal Builder1/1(Signal 1) -> MATLAB Function/2(wi)
  Signal Builder/1(Signal 1) -> MATLAB Function/1(wd)

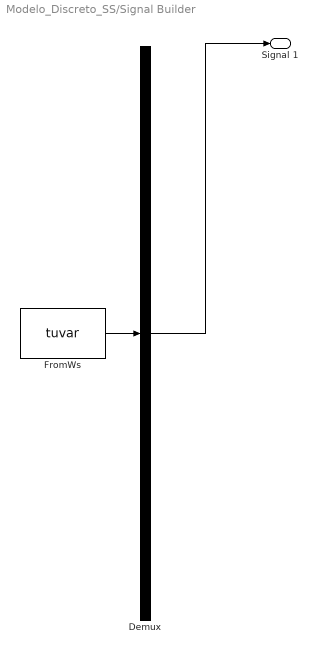
== system Modelo_Discreto_SS/Signal Builder ==
  Demux : Demux  Tag=STV Demux  Outputs=1
  FromWs : FromWorkspace  Tag=STV FromWs  VariableName=tuvar  SampleTime=0
      SigBuilderData=|
      | common.afterFinalStr = 'Extrapolate'
      | common.sampleTime = 0
      | dataSet.timeRange = [0 500]
      | dataSet.name = 'Group 1'
      | sbobj.Groups.Name = 'Group 1'
      | sbobj.Groups.Signals.Name = 'Signal 1'
      | sbobj.Groups.Signals.XData = [0 500]
      | sbobj.Groups.Signals.YData = [10 10]
      | sbobj.Groups.TimeRange = [0 500]
  Signal 1 : Outport  Tag=STV Outport
  wires:
  Demux/1 -> Signal 1/1
  FromWs/1 -> Demux/1

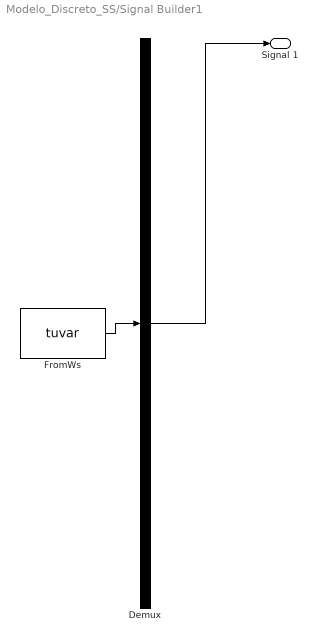
== system Modelo_Discreto_SS/Signal Builder1 ==
  Demux : Demux  Tag=STV Demux  Outputs=1
  FromWs : FromWorkspace  Tag=STV FromWs  VariableName=tuvar  SampleTime=0
      SigBuilderData=|
      | common.afterFinalStr = 'Extrapolate'
      | common.sampleTime = 0
      | dataSet.timeRange = [0 500]
      | dataSet.name = 'Group 1'
      | sbobj.Groups.Name = 'Group 1'
      | sbobj.Groups.Signals.Name = 'Signal 1'
      | sbobj.Groups.Signals.XData = [0 500]
      | sbobj.Groups.Signals.YData = [10 10]
      | sbobj.Groups.TimeRange = [0 500]
  Signal 1 : Outport  Tag=STV Outport
  wires:
  Demux/1 -> Signal 1/1
  FromWs/1 -> Demux/1

== matlab function Modelo_Discreto_SS/MATLAB Function1 ==
  data: x output; xk input; y output; yk input; thetak input; V_k input; w_k input; theta output; theta_k input
function [x,y,theta] = modelo_dis(xk,yk,thetak,V_k,w_k,theta_k)
Ts=0.5;
F=eye(3); %%matriz identidad
Fk= [xk;yk;thetak]; %% Las inicializamos en 0 ya que partimos desde el origen
B= [Ts*cos(theta_k) 0; Ts*sin(theta_k) 0; 0 Ts]; %%
u= [ V_k; w_k];

out = (Fk)+(B*u);
x=out(1);
y=out(2);
theta=out(3);

== matlab function Modelo_Discreto_SS/MATLAB Function ==
  data: theta output; wd input; V output; wi input; w output
function [theta,V,w] = pre_proceso(wd,wi)
r=0.625;
b=19.5;
vi= r*wi;
vd= r*wd;
V = (vd+vi)/2;
w = (wi-wd)/b;
theta = w*r;
